simulink model "DFIGPI_by_indraneel_saki"  (Simulink 10.0)
settings: Solver=ode23t  StartTime=0.0  StopTime=1.5  RelTol=1e-3  EnableMultiTasking=on
libraries: simulink x3, powerlib_extras x1, DRlib x1, powerlib x1
settings Model: Creator=SRIDHAR  LastModifiedBy=bhisma
settings SolverCC: ZeroCrossControl=DisableAll
settings DataIOCC: LimitDataPoints=on  SignalLoggingSaveFormat=ModelDataLogs
settings OptimizationCC: ExpressionDepthLimit=2147483647  InitFltsAndDblsToZero=on
settings DebuggingCC: SaveWithParameterizedLinksMsg=none  SignalResolutionControl=TryResolveAllWithWarning  SolverPrmCheckMsg=warning  FcnCallInpInsideContextMsg=warning  StateNameClashWarn=warning
settings GRTTargetCC: TargetFcnLib=ansi_tfl_tmw.mat  GeneratePreprocessorConditionals=Disable all
settings ConfigComp: CovExternalEMLEnable=off
settings SimscapeCC: SimscapeNormalizeSystem=off

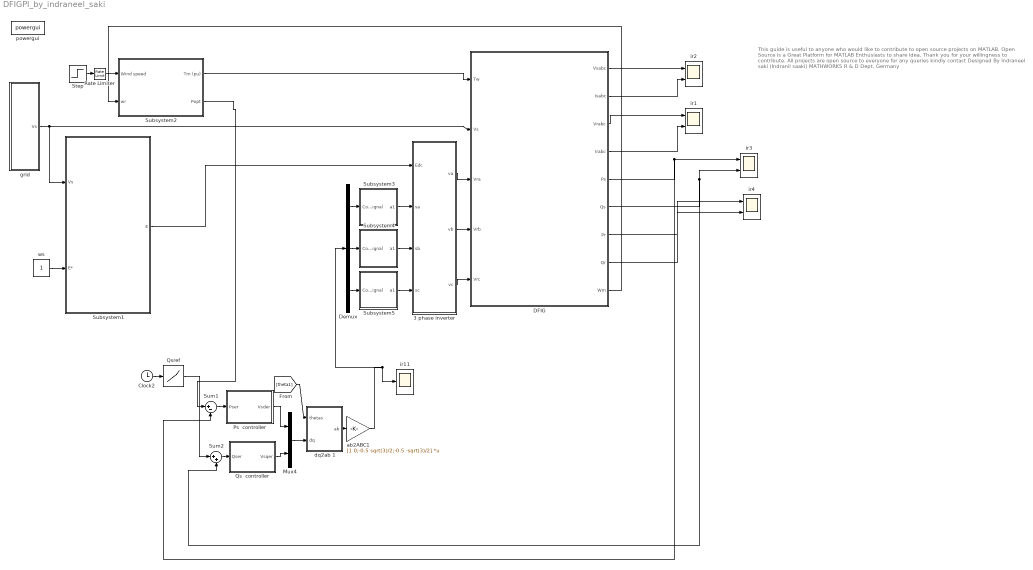
== system DFIGPI_by_indraneel_saki ==
  note: This guide is useful to anyone who would like to contribute to open source projects on MATLAB.
      | Open Source is a Great Platform for MATLAB Enthusiasts to share idea. Thank you for your willingness to contribute.
      | All projects are open source to everyone for any queries kindly contact
      | Designed By Indraneel saki (Indranil saaki)
      | MATHWORKS R & D Dept.
      | Germany
  3 phase inverter : Subsystem
  Clock2 : Clock
  DFIG : Subsystem
      mask Display: disp('DOUBLY FED\nINDUCTION\nGENERTATOR')
  Demux : Demux  Outputs=3
  Mux4 : Mux  Inputs=2
  Ps  controller : Subsystem  mask{Kp=0.07, Ki=10, sat=10}
      mask prompts: Kp "Proportional gain (Kp)"; Ki "Integral gain (Ki)"; sat "Saturation limit [pu]"
      mask help: Proportional-Integral Speed Controller
  Qs  controller : Subsystem  mask{Kp=0.07, Ki=10, sat=1000}
      mask prompts: Kp "Proportional gain (Kp)"; Ki "Integral gain (Ki)"; sat "Saturation limit [pu]"
      mask help: Proportional-Integral Speed Controller
  Qsref : Lookup  InputValues=[0 4 4 5]  Table=[1 1 4 1]  SaturateOnIntegerOverflow=on
  Rate Limiter : RateLimiter
  Step : Step  Time=5  Before=8  After=14  SampleTime=0
  Subsystem1 : Subsystem
      mask Display: disp('front end \n converter ')
  Subsystem2 : Subsystem  mask{speed_power=[0 0; 0.24 0.007; 0.36 0.024; 0.6 0.112; 0.96 0.46; 1.2 0.898; 1.5 0.898], speed_ABCD=[0.7 0.71 1.2 1.21], power_slew_rate=1, pitch_rate=2, pitch_max=45, pitch_gain=500}
      mask prompts: speed_power "Electric power-speed characteristic: [wr1(pu) p1(pu); wr2(pu) p2(pu); ... ]"; speed_ABCD "Tracking characteristic speeds: [speed_A(pu) ... speed_D(pu)]"; power_slew_rate "Maximum rate of change of reference power (p.u./s):"; pitch_rate "Maximum rate of change of pitch angle (deg/s):"; pitch_max "Maximum pitch angle (deg):"; pitch_gain "Pitch angle controller gain [Kp]:"
      mask Display: disp('Wind\nTurbine')
  Subsystem3 : Subsystem  mask{fs=2000}
      mask prompts: fs "Switching Frequency"
  Subsystem4 : Subsystem  mask{fs=2000}
      mask prompts: fs "Switching Frequency"
  Subsystem5 : Subsystem  mask{fs=2000}
      mask prompts: fs "Switching Frequency"
  Sum1 : Sum  Inputs=|+-  SaturateOnIntegerOverflow=on
  Sum2 : Sum  Inputs=|++  SaturateOnIntegerOverflow=on
  ab2ABC1 : Gain  Gain=[1 0;-0.5 sqrt(3)/2;-0.5 -sqrt(3)/2]  Multiplication=Matrix(K*u)  SaturateOnIntegerOverflow=on  OutDataTypeStr=Inherit: Same as input  ParamDataTypeStr=Inherit: Same as input
  dq2ab 1 : Subsystem
  grid : Subsystem
      mask Display: disp('GRID')
  ir{1..4} (4 alike) : Scope  NumInputPorts=2
  ir11 : Scope
  powergui : powerlib/powergui  SystemSampleTime=-1  SimulationMode=Continuous  SampleTime=50e-6  frequency=60  SPID=off  DisableSnubberDevices=off  DisableRonSwitches=off  DisableVfSwitches=off  SwTol=0  Interpol=off  frequencyindice=0  echomessages=off  HookPort=off  DisplayEquations=off  FunctionMessages=off  EnableUseOfTLC=off  x0status=blocks  RestoreLinks=warning  Frange=[0:2:500]  Ylog=off  Xlog=on  ShowGrid=off  save=off  variable=ZData  ZoomFFT=on  StartTime=0.0  cycles=1  DisplayStyle=1  fundamental=60  FreqAxis=off  MaxFrequency=1000  frequencyindicesteady=1  RmsSteady=1  display=off  Ts=0  methode=off
      settings: SourceProductName=Simscape Electrical
  ws : Constant
  wires:
  grid/1(Vs) -> Subsystem1/1(Vs), DFIG/2(Vs)
  3 phase inverter/1(va) -> DFIG/3(Vra)
  3 phase inverter/2(vb) -> DFIG/4(Vrb)
  3 phase inverter/3(vc) -> DFIG/5(Vrc)
  DFIG/1(Vsabc) -> ir2/1
  DFIG/2(Isabc) -> ir2/2
  DFIG/3(Vrabc) -> ir1/1
  DFIG/4(Irabc) -> ir1/2
  Demux/3 -> Subsystem5/1(Control signal)
  Demux/1 -> Subsystem3/1(Control signal)
  Demux/2 -> Subsystem4/1(Control signal)
  Subsystem1/1(E) -> 3 phase inverter/1(Edc)
  ws/1 -> Subsystem1/2("E* ")
  DFIG/7(Pr) -> ir4/1
  DFIG/8(Qr) -> ir4/2
  DFIG/5(Ps) -> Sum1/2, ir3/1
  DFIG/6(Qs) -> Sum2/2, ir3/2
  Qsref/1 -> Sum2/1
  Subsystem2/1(Tm (pu)) -> DFIG/1(Tw)
  Subsystem2/2(Popt) -> Sum1/1
  DFIG/9(Wm) -> Subsystem2/2(wr)
  Step/1 -> Rate Limiter/1
  Sum1/1 -> Ps  controller/1(Pser)
  Sum2/1 -> Qs  controller/1(Qser)
  Ps  controller/1(Vsder) -> Mux4/1
  Qs  controller/1(Vsqer) -> Mux4/2
  Mux4/1 -> dq2ab 1/2(dq)
  dq2ab 1/1(ab) -> ab2ABC1/1
  ab2ABC1/1 -> Demux/1, ir11/1
  [theta1] -> dq2ab 1/1(thetas)
  Clock2/1 -> Qsref/1
  Subsystem3/1(a1) -> 3 phase inverter/2(sa)
  Subsystem4/1(a1) -> 3 phase inverter/3(sb)
  Subsystem5/1(a1) -> 3 phase inverter/4(sc)
  Rate Limiter/1 -> Subsystem2/1("Wind speed ")

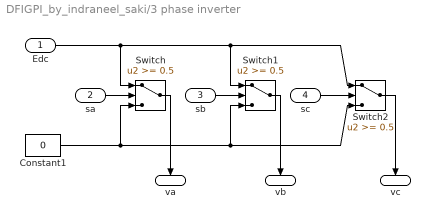
== system DFIGPI_by_indraneel_saki/3 phase inverter ==
  Edc : Inport
  sa : Inport  Port=2
  sb : Inport  Port=3
  sc : Inport  Port=4
  Constant1 : Constant  Value=0
  Switch : Switch  Threshold=0.5  SaturateOnIntegerOverflow=on  InputSameDT=on
  Switch1 : Switch  Threshold=0.5  SaturateOnIntegerOverflow=on  InputSameDT=on
  Switch2 : Switch  Threshold=0.5  SaturateOnIntegerOverflow=on  InputSameDT=on
  va : Outport  InitialOutput=0
  vb : Outport  Port=2  InitialOutput=0
  vc : Outport  Port=3  InitialOutput=0
  wires:
  Switch1/1 -> vb/1
  Switch2/1 -> vc/1
  sc/1 -> Switch2/2
  sb/1 -> Switch1/2
  Switch/1 -> va/1
  sa/1 -> Switch/2
  Constant1/1 -> Switch2/3, Switch1/3, Switch/3
  Edc/1 -> Switch2/1, Switch1/1, Switch/1

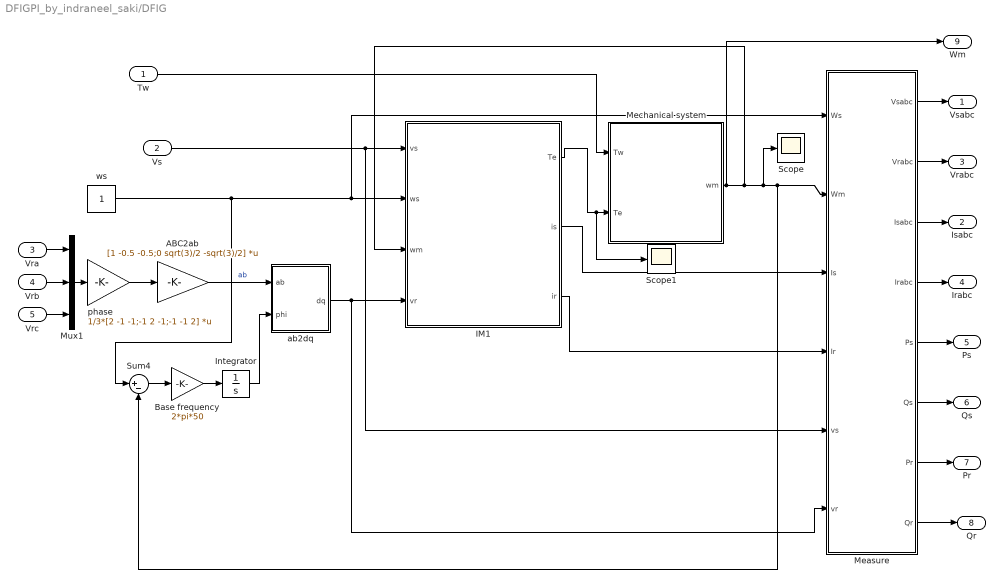
== system DFIGPI_by_indraneel_saki/DFIG ==
  Tw : Inport
  Vs : Inport  Port=2
  Vra : Inport  Port=3
  Vrb : Inport  Port=4
  Vrc : Inport  Port=5
  ABC2ab : Gain  Gain=[1 -0.5 -0.5;0 sqrt(3)/2 -sqrt(3)/2]  Multiplication=Matrix(K*u)  SaturateOnIntegerOverflow=on  OutDataTypeStr=Inherit: Same as input  ParamDataTypeStr=Inherit: Same as input
  Base frequency : Gain  Gain=2*pi*50  SaturateOnIntegerOverflow=on  OutDataTypeStr=Inherit: Same as input  ParamDataTypeStr=Inherit: Same as input
  IM1 : Subsystem  mask{Rs=0.05, Lsl=0.5, Rr=0.02, Lm=5, Lrl=0.1, wo=100*pi}
      mask prompts: Rs "Stator resistance [pu]"; Lsl "Stator leakage inductance [pu]"; Rr "Rotor resistance [pu]"; Lm "Magnetizing inductance [pu]"; Lrl "Rotor leakage inductance [pu]"; wo "base frequency [rad/s]"
      mask Display: disp('DOUBLY FED\nINDUCTION GENERTATOR')
  Integrator : Integrator
  Measure : Subsystem
  Mechanical system : Subsystem  mask{Hw=2.5, Hg=0.5, Km=.4}
      mask prompts: Hw "Turbine inertia constant [s]"; Hg "Generator inertia constant [s]"; Km "Shaft compliance constant [pu/rad]"
      mask Display: disp('Mechanical\nSystem')
  Mux1 : Mux  Inputs=3
  Scope : Scope
  Scope1 : Scope
  Sum4 : Sum  Inputs=|+-  SaturateOnIntegerOverflow=on  InputSameDT=on  OutDataTypeStr=Inherit: Same as first input
  ab2dq : Subsystem
  phase : Gain  Gain=1/3*[2 -1 -1;-1 2 -1;-1 -1 2]  Multiplication=Matrix(K*u)  SaturateOnIntegerOverflow=on  OutDataTypeStr=Inherit: Same as input  ParamDataTypeStr=Inherit: Same as input
  ws : Constant
  Vsabc : Outport
  Isabc : Outport  Port=2
  Vrabc : Outport  Port=3
  Irabc : Outport  Port=4
  Ps : Outport  Port=5
  Qs : Outport  Port=6
  Pr : Outport  Port=7
  Qr : Outport  Port=8
  Wm : Outport  Port=9
  wires:
  Vra/1 -> Mux1/1
  Vrb/1 -> Mux1/2
  Vrc/1 -> Mux1/3
  Mux1/1 -> phase/1
  Measure/1(Vsabc) -> Vsabc/1
  Measure/2(Vrabc) -> Vrabc/1
  Measure/3(Isabc) -> Isabc/1
  Measure/4(Irabc) -> Irabc/1
  Measure/5(Ps) -> Ps/1
  Measure/6(Qs) -> Qs/1
  phase/1 -> ABC2ab/1
  Mechanical system/1(wm) -> Wm/1, IM1/3(wm), Measure/2(Wm), Sum4/2, Scope/1
  IM1/1(Te) -> Mechanical system/2(Te), Scope1/1
  Tw/1 -> Mechanical system/1(Tw)
  ws/1 -> Measure/1(Ws), IM1/2(ws), Sum4/1
  Vs/1 -> IM1/1(vs), Measure/5(vs)
  IM1/2(is) -> Measure/3(Is)
  IM1/3(ir) -> Measure/4(Ir)
  Measure/7(Pr) -> Pr/1
  Measure/8(Qr) -> Qr/1
  ABC2ab/1 -> ab2dq/1(ab)  "ab"
  Base frequency/1 -> Integrator/1
  Integrator/1 -> ab2dq/2(phi)
  Sum4/1 -> Base frequency/1
  ab2dq/1(dq) -> IM1/4(vr), Measure/6(vr)

== system DFIGPI_by_indraneel_saki/Ps  controller ==
  Pser : Inport
  Gain : Gain  Gain=Ki  SaturateOnIntegerOverflow=on  OutDataTypeStr=Inherit: Same as input  ParamDataTypeStr=Inherit: Same as input
  Gain1 : Gain  Gain=Kp  SaturateOnIntegerOverflow=on  OutDataTypeStr=Inherit: Same as input  ParamDataTypeStr=Inherit: Same as input
  Integrator : Integrator  LimitOutput=on  UpperSaturationLimit=sat  LowerSaturationLimit=-sat
  Saturation : Saturate  UpperLimit=sat  LowerLimit=-sat
  Sum : Sum  SaturateOnIntegerOverflow=on  InputSameDT=on  OutDataTypeStr=Inherit: Same as first input
  Vsder : Outport  InitialOutput=0
  wires:
  Integrator/1 -> Sum/2
  Gain1/1 -> Sum/1
  Gain/1 -> Integrator/1
  Pser/1 -> Gain/1, Gain1/1
  Sum/1 -> Saturation/1
  Saturation/1 -> Vsder/1

== system DFIGPI_by_indraneel_saki/Qs  controller ==
  Qser : Inport
  Gain : Gain  Gain=Ki  SaturateOnIntegerOverflow=on  OutDataTypeStr=Inherit: Same as input  ParamDataTypeStr=Inherit: Same as input
  Gain1 : Gain  Gain=Kp  SaturateOnIntegerOverflow=on  OutDataTypeStr=Inherit: Same as input  ParamDataTypeStr=Inherit: Same as input
  Integrator : Integrator  LimitOutput=on  UpperSaturationLimit=sat  LowerSaturationLimit=-sat
  Saturation : Saturate  UpperLimit=sat  LowerLimit=-sat
  Sum : Sum  SaturateOnIntegerOverflow=on  InputSameDT=on  OutDataTypeStr=Inherit: Same as first input
  Vsqer : Outport  InitialOutput=0
  wires:
  Saturation/1 -> Vsqer/1
  Sum/1 -> Saturation/1
  Qser/1 -> Gain1/1, Gain/1
  Gain/1 -> Integrator/1
  Gain1/1 -> Sum/1
  Integrator/1 -> Sum/2

== system DFIGPI_by_indraneel_saki/Subsystem1 ==
  Vs : Inport
  "E* " : Inport  Port=2
  Ps  controller : Subsystem  mask{Kp=0.07, Ki=10, sat=1000}
      mask prompts: Kp "Proportional gain (Kp)"; Ki "Integral gain (Ki)"; sat "Saturation limit [pu]"
      mask help: Proportional-Integral Speed Controller
  Subsystem : Subsystem
      mask Display: disp('INVERTER')
  Sum : Sum  Inputs=|+-
  Transfer Fcn : TransferFcn  Denominator=[2.4e-6 0]
  E : Outport
  wires:
  Transfer Fcn/1 -> Sum/2, E/1
  "E* "/1 -> Sum/1, Subsystem/2("E* ")
  Sum/1 -> Ps  controller/1(Pser)
  Subsystem/1(Ios) -> Transfer Fcn/1
  Vs/1 -> Subsystem/1(Vs)
  Ps  controller/1(Vsder) -> Subsystem/3(Id)

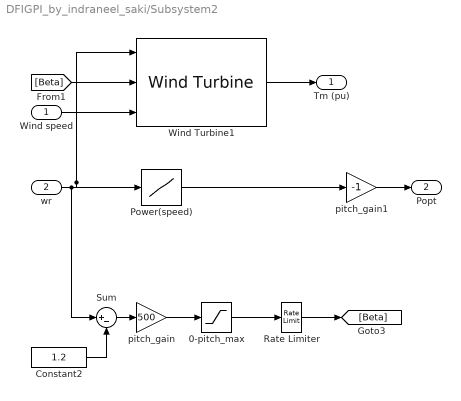
== system DFIGPI_by_indraneel_saki/Subsystem2 ==
  "Wind speed " : Inport
  wr : Inport  Port=2
  0-pitch_max : Saturate  UpperLimit=pitch_max  LowerLimit=0
  Constant2 : Constant  Value=1.2
  Power(speed) : Lookup  InputValues=speed_power(:,1)  Table=speed_power(:,2)  SaturateOnIntegerOverflow=on
  "Rate Limiter   " : RateLimiter  RisingSlewLimit=pitch_rate  FallingSlewLimit=-pitch_rate
  Sum : Sum  Inputs=|+-  SaturateOnIntegerOverflow=on
  Wind Turbine1 : DRlib/Wind Generation/Wind Turbine  SystemSampleTime=-1  Pnom=1.5e6  Pelec_base=1.5e6/0.9  wind_base=12  P_wind_base=0.73  speed_nom=1.2  pitch_angle=0  DisplayTurbChar=off  c1_c6="[0.51763          116          0.4            5           21     0.006795]"  cp_nom=0.48  lambda_nom=8.1
      settings: SourceProductName=Simscape Electrical  SourceProductBaseCode=PS
  pitch_gain : Gain  Gain=500  SaturateOnIntegerOverflow=on  OutDataTypeStr=Inherit: Same as input  ParamDataTypeStr=Inherit: Same as input
  pitch_gain1 : Gain  Gain=-1  SaturateOnIntegerOverflow=on  OutDataTypeStr=Inherit: Same as input  ParamDataTypeStr=Inherit: Same as input
  Tm (pu) : Outport
  Popt : Outport  Port=2
  wires:
  wr/1 -> Sum/1, Wind Turbine1/1, Power(speed)/1
  pitch_gain/1 -> 0-pitch_max/1
  Sum/1 -> pitch_gain/1
  Constant2/1 -> Sum/2
  [Beta] -> Wind Turbine1/2
  Wind Turbine1/1 -> Tm (pu)/1
  "Wind speed "/1 -> Wind Turbine1/3
  Power(speed)/1 -> pitch_gain1/1
  pitch_gain1/1 -> Popt/1
  "Rate Limiter   "/1 -> [Beta]
  0-pitch_max/1 -> "Rate Limiter   "/1

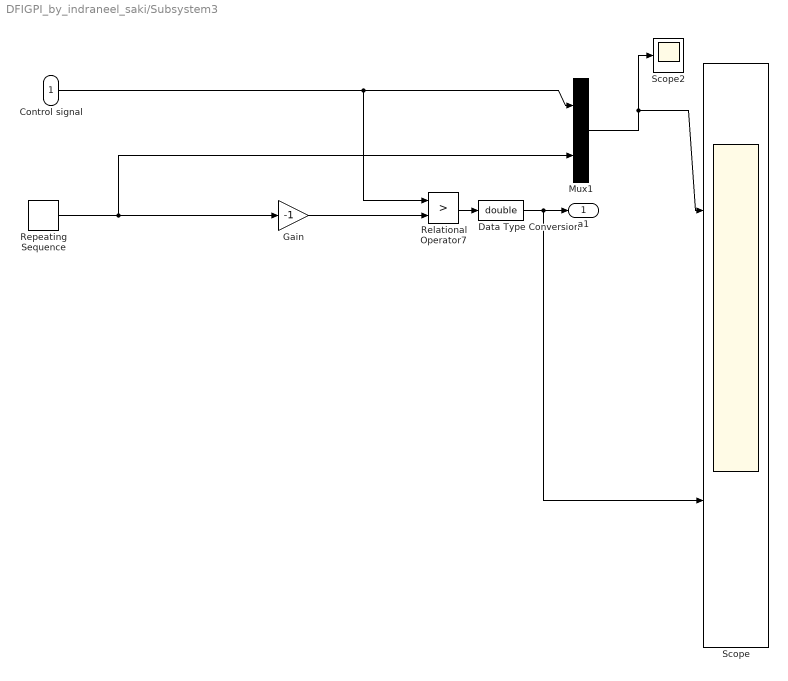
== system DFIGPI_by_indraneel_saki/Subsystem3 ==
  Control signal : Inport
  Data Type Conversion : DataTypeConversion  OutDataTypeStr=double
  Gain : Gain  Gain=-1
  Mux1 : Mux  Inputs=2
  Relational Operator7 : RelationalOperator  Operator=>  OutDataTypeStr=uint(8)  RndMeth=Nearest
  Repeating Sequence : simulink/Sources/Repeating Sequence  SystemSampleTime=-1  rep_seq_t=[0 (1/fs)/2 1/fs]  rep_seq_y=[1 -1 1 ]
  Scope : Scope  NumInputPorts=2
  Scope2 : Scope
  a1 : Outport
  wires:
  Repeating Sequence/1 -> Mux1/2, Gain/1
  Relational Operator7/1 -> Data Type Conversion/1
  Control signal/1 -> Mux1/1, Relational Operator7/1
  Data Type Conversion/1 -> a1/1, Scope/2
  Gain/1 -> Relational Operator7/2
  Mux1/1 -> Scope/1, Scope2/1

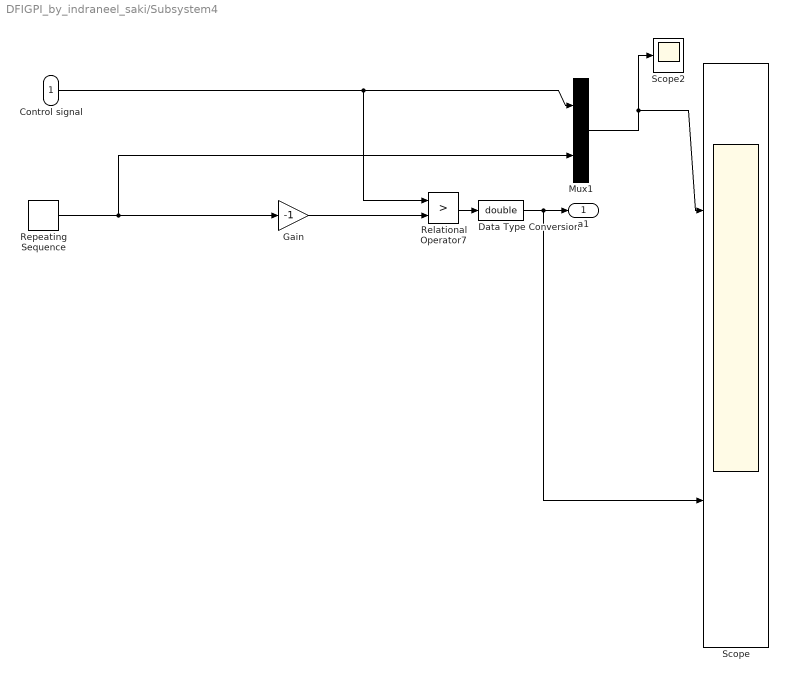
== system DFIGPI_by_indraneel_saki/Subsystem4 ==
  Control signal : Inport
  Data Type Conversion : DataTypeConversion  OutDataTypeStr=double
  Gain : Gain  Gain=-1
  Mux1 : Mux  Inputs=2
  Relational Operator7 : RelationalOperator  Operator=>  OutDataTypeStr=uint(8)  RndMeth=Nearest
  Repeating Sequence : simulink/Sources/Repeating Sequence  SystemSampleTime=-1  rep_seq_t=[0 (1/fs)/2 1/fs]  rep_seq_y=[1 -1 1 ]
  Scope : Scope  NumInputPorts=2
  Scope2 : Scope
  a1 : Outport
  wires:
  Mux1/1 -> Scope2/1, Scope/1
  Gain/1 -> Relational Operator7/2
  Data Type Conversion/1 -> Scope/2, a1/1
  Control signal/1 -> Relational Operator7/1, Mux1/1
  Relational Operator7/1 -> Data Type Conversion/1
  Repeating Sequence/1 -> Gain/1, Mux1/2

== system DFIGPI_by_indraneel_saki/Subsystem5 ==
  Control signal : Inport
  Data Type Conversion : DataTypeConversion  OutDataTypeStr=double
  Gain : Gain  Gain=-1
  Mux1 : Mux  Inputs=2
  Relational Operator7 : RelationalOperator  Operator=>  OutDataTypeStr=uint(8)  RndMeth=Nearest
  Repeating Sequence : simulink/Sources/Repeating Sequence  SystemSampleTime=-1  rep_seq_t=[0 (1/fs)/2 1/fs]  rep_seq_y=[1 -1 1 ]
  Scope : Scope  NumInputPorts=2
  Scope2 : Scope
  a1 : Outport
  wires:
  Repeating Sequence/1 -> Mux1/2, Gain/1
  Relational Operator7/1 -> Data Type Conversion/1
  Control signal/1 -> Mux1/1, Relational Operator7/1
  Data Type Conversion/1 -> a1/1, Scope/2
  Gain/1 -> Relational Operator7/2
  Mux1/1 -> Scope/1, Scope2/1

== system DFIGPI_by_indraneel_saki/dq2ab 1 ==
  thetas : Inport
  dq : Inport  Port=2
  Fcn : Fcn  Expr=u(1)*cos(u(3))-u(2)*sin(u(3))
  Fcn1 : Fcn  Expr=u(1)*sin(u(3))+u(2)*cos(u(3))
  Mux3 : Mux  Inputs=2
  Mux4 : Mux  Inputs=2
  Mux5 : Mux  Inputs=2
  ab : Outport
  wires:
  Mux5/1 -> ab/1
  Fcn/1 -> Mux5/1
  Fcn1/1 -> Mux5/2
  thetas/1 -> Mux4/2, Mux3/2
  dq/1 -> Mux4/1, Mux3/1
  Mux4/1 -> Fcn1/1
  Mux3/1 -> Fcn/1

== system DFIGPI_by_indraneel_saki/grid ==
  note: Vds
  note: Vqs
  Mux3 : Mux  Inputs=2
  Vds : Constant
  vqs : Constant  Value=0
  Vs : Outport
  wires:
  Mux3/1 -> Vs/1
  Vds/1 -> Mux3/1
  vqs/1 -> Mux3/2

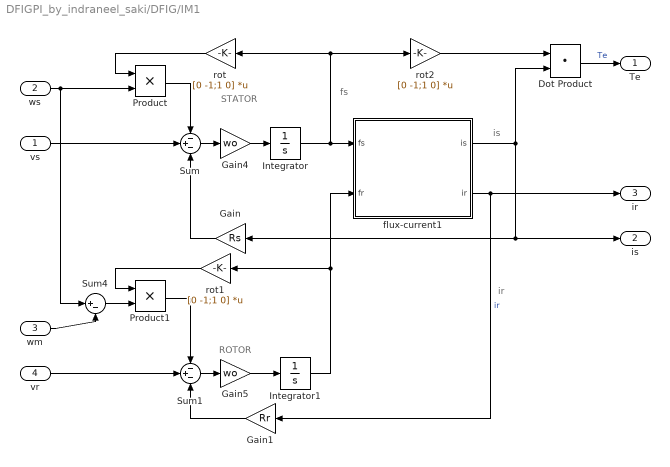
== system DFIGPI_by_indraneel_saki/DFIG/IM1 ==
  note: fs
  note: is
  note: ir
  note: ROTOR
  note: STATOR
  vs : Inport
  ws : Inport  Port=2
  wm : Inport  Port=3
  vr : Inport  Port=4
  Dot Product : DotProduct  InputSameDT=on  OutDataTypeStr=Inherit: Inherit via internal rule
  Gain : Gain  Gain=Rs  SaturateOnIntegerOverflow=on  OutDataTypeStr=Inherit: Same as input  ParamDataTypeStr=Inherit: Same as input
  Gain1 : Gain  Gain=Rr  SaturateOnIntegerOverflow=on  OutDataTypeStr=Inherit: Same as input  ParamDataTypeStr=Inherit: Same as input
  Gain4 : Gain  Gain=wo  SaturateOnIntegerOverflow=on  OutDataTypeStr=Inherit: Same as input  ParamDataTypeStr=Inherit: Same as input
  Gain5 : Gain  Gain=wo  SaturateOnIntegerOverflow=on  OutDataTypeStr=Inherit: Same as input  ParamDataTypeStr=Inherit: Same as input
  Integrator : Integrator
  Integrator1 : Integrator
  Product : Product  SaturateOnIntegerOverflow=on  InputSameDT=on  OutDataTypeStr=Inherit: Same as first input
  Product1 : Product  SaturateOnIntegerOverflow=on  InputSameDT=on  OutDataTypeStr=Inherit: Same as first input
  Sum : Sum  Inputs=-+-  SaturateOnIntegerOverflow=on  InputSameDT=on  OutDataTypeStr=Inherit: Same as first input
  Sum1 : Sum  Inputs=-+-  SaturateOnIntegerOverflow=on  InputSameDT=on  OutDataTypeStr=Inherit: Same as first input
  Sum4 : Sum  Inputs=|+-  SaturateOnIntegerOverflow=on  InputSameDT=on  OutDataTypeStr=Inherit: Same as first input
  flux-current1 : Subsystem
  rot : Gain  Gain=[0 -1;1 0]  Multiplication=Matrix(K*u)  SaturateOnIntegerOverflow=on  OutDataTypeStr=Inherit: Same as input  ParamDataTypeStr=Inherit: Same as input
  rot1 : Gain  Gain=[0 -1;1 0]  Multiplication=Matrix(K*u)  SaturateOnIntegerOverflow=on  OutDataTypeStr=Inherit: Same as input  ParamDataTypeStr=Inherit: Same as input
  rot2 : Gain  Gain=[0 -1;1 0]  Multiplication=Matrix(K*u)  SaturateOnIntegerOverflow=on  OutDataTypeStr=Inherit: Same as input  ParamDataTypeStr=Inherit: Same as input
  Te : Outport
  is : Outport  Port=2
  ir : Outport  Port=3
  wires:
  Gain/1 -> Sum/3
  Gain1/1 -> Sum1/3
  flux-current1/2(ir) -> Gain1/1, ir/1  "ir"
  Integrator/1 -> flux-current1/1(fs), rot/1, rot2/1
  Integrator1/1 -> flux-current1/2(fr), rot1/1
  Product1/1 -> Sum1/1
  rot1/1 -> Product1/1
  Product/1 -> Sum/1
  rot/1 -> Product/1
  rot2/1 -> Dot Product/1
  Sum4/1 -> Product1/2
  Sum/1 -> Gain4/1
  Gain4/1 -> Integrator/1
  Sum1/1 -> Gain5/1
  Gain5/1 -> Integrator1/1
  flux-current1/1(is) -> Gain/1, is/1, Dot Product/2
  Dot Product/1 -> Te/1  "Te"
  vs/1 -> Sum/2
  ws/1 -> Product/2, Sum4/1
  wm/1 -> Sum4/2
  vr/1 -> Sum1/2

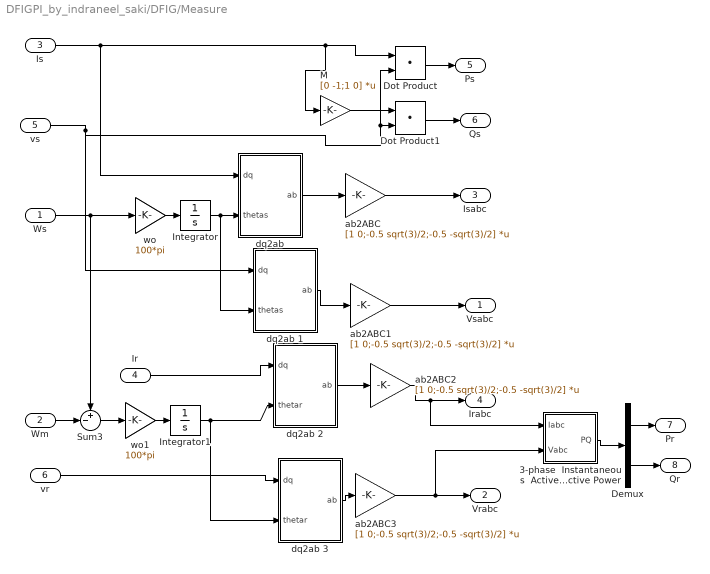
== system DFIGPI_by_indraneel_saki/DFIG/Measure ==
  Ws : Inport
  Wm : Inport  Port=2
  Is : Inport  Port=3
  Ir : Inport  Port=4
  vs : Inport  Port=5
  vr : Inport  Port=6
  3-phase  Instantaneous  Active & Reactive Power : Subsystem  AncestorBlock=|  DialogController=PMDialogs.PMDefaultMaskDlg  mask(3-phase instantaneous active and reactive power){}
      | powerlib_extras/Measurements/3-phase 
      | Instantaneous 
      | Active & Reactive Power
      mask help:
      | This block computes the 3-phase instantaneous active (P) and reactive (Q) power associated with a periodic set of 3-phase voltages and currents.
      | Note: Result for the instantaneous reactive power (Q) is accurate only for balanced and harmonic-free 3-phase quantities (voltages and currents).
      |
      | Input 1: Vectorized 3-phase  instantaneous voltage (Vabc)
      | Input 2: Vectorized 3-phase instantaneous current (Iabc)
      | Output : Computed PQ vector [P(W) Q(var)]. Current flowing into an RL circuit will produce  positive active and reactive power.
      mask init:
      | power_initmask();
      mask Help: This block is part of a subset of blocks in the Extras library that does not have documentation associated with it, other than the block mask description.
  Demux : Demux  Outputs=2
  Dot Product : DotProduct  InputSameDT=on  OutDataTypeStr=Inherit: Inherit via internal rule
  Dot Product1 : DotProduct  InputSameDT=on  OutDataTypeStr=Inherit: Inherit via internal rule
  Integrator : Integrator
  Integrator1 : Integrator
  M : Gain  Gain=[0 -1;1 0]  Multiplication=Matrix(K*u)  SaturateOnIntegerOverflow=on  OutDataTypeStr=Inherit: Same as input  ParamDataTypeStr=Inherit: Same as input
  Sum3 : Sum  Inputs=+-|  SaturateOnIntegerOverflow=on
  ab2ABC{,1..3} (4 alike) : Gain  Gain=[1 0;-0.5 sqrt(3)/2;-0.5 -sqrt(3)/2]  Multiplication=Matrix(K*u)  SaturateOnIntegerOverflow=on  OutDataTypeStr=Inherit: Same as input  ParamDataTypeStr=Inherit: Same as input
  "dq2ab " : Subsystem
  dq2ab 1 : Subsystem
  dq2ab 2 : Subsystem
  dq2ab 3 : Subsystem
  wo : Gain  Gain=100*pi  SaturateOnIntegerOverflow=on  OutDataTypeStr=Inherit: Same as input  ParamDataTypeStr=Inherit: Same as input
  wo1 : Gain  Gain=100*pi  SaturateOnIntegerOverflow=on  OutDataTypeStr=Inherit: Same as input  ParamDataTypeStr=Inherit: Same as input
  Vsabc : Outport
  Vrabc : Outport  Port=2
  Isabc : Outport  Port=3
  Irabc : Outport  Port=4
  Ps : Outport  Port=5
  Qs : Outport  Port=6
  Pr : Outport  Port=7
  Qr : Outport  Port=8
  wires:
  Is/1 -> "dq2ab "/1(dq), M/1, Dot Product/1
  vs/1 -> dq2ab 1/1(dq), Dot Product/2, Dot Product1/2
  Ir/1 -> dq2ab 2/1(dq)
  vr/1 -> dq2ab 3/1(dq)
  "dq2ab "/1(ab) -> ab2ABC/1
  ab2ABC/1 -> Isabc/1
  wo/1 -> Integrator/1
  Integrator/1 -> "dq2ab "/2(thetas), dq2ab 1/2(thetas)
  Ws/1 -> Sum3/1, wo/1
  dq2ab 1/1(ab) -> ab2ABC1/1
  ab2ABC1/1 -> Vsabc/1
  Wm/1 -> Sum3/2
  Sum3/1 -> wo1/1
  wo1/1 -> Integrator1/1
  dq2ab 2/1(ab) -> ab2ABC2/1
  ab2ABC2/1 -> Irabc/1, 3-phase  Instantaneous  Active & Reactive Power/1(Iabc)
  Integrator1/1 -> dq2ab 2/2(thetar), dq2ab 3/2(thetar)
  dq2ab 3/1(ab) -> ab2ABC3/1
  ab2ABC3/1 -> Vrabc/1, 3-phase  Instantaneous  Active & Reactive Power/2(Vabc)
  Dot Product/1 -> Ps/1
  Dot Product1/1 -> Qs/1
  M/1 -> Dot Product1/1
  3-phase  Instantaneous  Active & Reactive Power/1(PQ) -> Demux/1
  Demux/1 -> Pr/1
  Demux/2 -> Qr/1

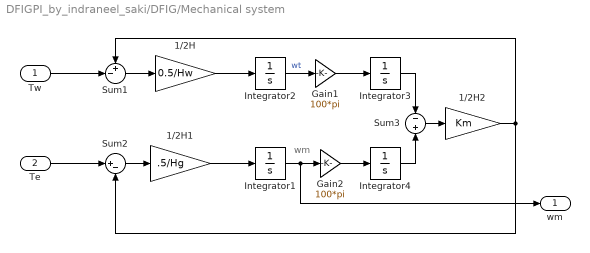
== system DFIGPI_by_indraneel_saki/DFIG/Mechanical system ==
  note: wm
  Tw : Inport
  Te : Inport  Port=2
  1/2H : Gain  Gain=0.5/Hw  SaturateOnIntegerOverflow=on  OutDataTypeStr=Inherit: Same as input  ParamDataTypeStr=Inherit: Same as input
  1/2H1 : Gain  Gain=.5/Hg  SaturateOnIntegerOverflow=on  OutDataTypeStr=Inherit: Same as input  ParamDataTypeStr=Inherit: Same as input
  1/2H2 : Gain  Gain=Km  SaturateOnIntegerOverflow=on  OutDataTypeStr=Inherit: Same as input  ParamDataTypeStr=Inherit: Same as input
  Gain1 : Gain  Gain=100*pi  SaturateOnIntegerOverflow=on  OutDataTypeStr=Inherit: Same as input  ParamDataTypeStr=Inherit: Same as input
  Gain2 : Gain  Gain=100*pi  SaturateOnIntegerOverflow=on  OutDataTypeStr=Inherit: Same as input  ParamDataTypeStr=Inherit: Same as input
  Integrator{1..4} (4 alike) : Integrator
  Sum1 : Sum  Inputs=+-|  SaturateOnIntegerOverflow=on
  Sum2 : Sum  Inputs=|+-  SaturateOnIntegerOverflow=on
  Sum3 : Sum  Inputs=-+  SaturateOnIntegerOverflow=on
  wm : Outport
  wires:
  Tw/1 -> Sum1/2
  Sum1/1 -> 1/2H/1
  Te/1 -> Sum2/1
  1/2H/1 -> Integrator2/1
  Sum2/1 -> 1/2H1/1
  1/2H1/1 -> Integrator1/1
  Integrator3/1 -> Sum3/1
  Sum3/1 -> 1/2H2/1
  1/2H2/1 -> Sum1/1, Sum2/2
  Gain1/1 -> Integrator3/1
  Integrator2/1 -> Gain1/1  "wt"
  Gain2/1 -> Integrator4/1
  Integrator4/1 -> Sum3/2
  Integrator1/1 -> Gain2/1, wm/1

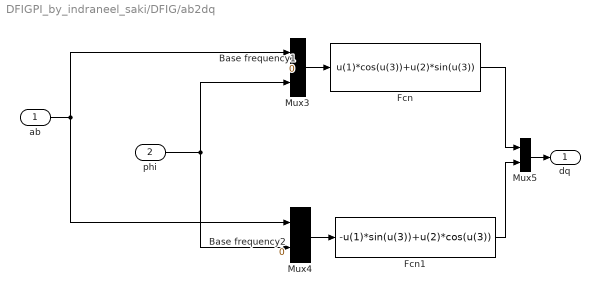
== system DFIGPI_by_indraneel_saki/DFIG/ab2dq ==
  ab : Inport
  phi : Inport  Port=2
  Base frequency1 : Gain  Gain=0  SaturateOnIntegerOverflow=on  OutDataTypeStr=Inherit: Same as input  ParamDataTypeStr=Inherit: Same as input
  Base frequency2 : Gain  Gain=0  SaturateOnIntegerOverflow=on  OutDataTypeStr=Inherit: Same as input  ParamDataTypeStr=Inherit: Same as input
  Fcn : Fcn  Expr=u(1)*cos(u(3))+u(2)*sin(u(3))
  Fcn1 : Fcn  Expr=-u(1)*sin(u(3))+u(2)*cos(u(3))
  Mux3 : Mux  Inputs=2
  Mux4 : Mux  Inputs=2
  Mux5 : Mux  Inputs=2
  dq : Outport
  wires:
  Mux3/1 -> Fcn/1
  Mux4/1 -> Fcn1/1
  ab/1 -> Mux3/1, Mux4/1
  Fcn1/1 -> Mux5/2
  Fcn/1 -> Mux5/1
  Mux5/1 -> dq/1
  phi/1 -> Base frequency1/1, Base frequency2/1
  Base frequency1/1 -> Mux3/2
  Base frequency2/1 -> Mux4/2

== system DFIGPI_by_indraneel_saki/Subsystem1/Ps  controller ==
  Pser : Inport
  Gain : Gain  Gain=Ki  SaturateOnIntegerOverflow=on  OutDataTypeStr=Inherit: Same as input  ParamDataTypeStr=Inherit: Same as input
  Gain1 : Gain  Gain=Kp  SaturateOnIntegerOverflow=on  OutDataTypeStr=Inherit: Same as input  ParamDataTypeStr=Inherit: Same as input
  Integrator : Integrator  LimitOutput=on  UpperSaturationLimit=sat  LowerSaturationLimit=-sat
  Saturation : Saturate  UpperLimit=sat  LowerLimit=-sat
  Sum : Sum  SaturateOnIntegerOverflow=on  InputSameDT=on  OutDataTypeStr=Inherit: Same as first input
  Vsder : Outport  InitialOutput=0
  wires:
  Integrator/1 -> Sum/2
  Gain1/1 -> Sum/1
  Pser/1 -> Gain/1, Gain1/1
  Sum/1 -> Saturation/1
  Saturation/1 -> Vsder/1
  Gain/1 -> Integrator/1

== system DFIGPI_by_indraneel_saki/Subsystem1/Subsystem ==
  note: M1
  Vs : Inport
  "E* " : Inport  Port=2
  Id : Inport  Port=3
  3M1/(2root2)1 : Gain  Gain=2*sqrt(2)/(3*sqrt(3))
  3M1/(2root2)2 : Gain  Gain=2*sqrt(2)/(3*sqrt(3))
  Divide : Product  Inputs=*/
  Fcn : Fcn  Expr=sqrt((u(1))^2 +((u(2))^2))
  Product : Product  RndMeth=Zero
  Ios : Outport
  wires:
  "E* "/1 -> Divide/2
  Vs/1 -> Fcn/1
  Fcn/1 -> Divide/1
  Divide/1 -> 3M1/(2root2)1/1
  3M1/(2root2)1/1 -> Product/1
  3M1/(2root2)2/1 -> Product/2
  Product/1 -> Ios/1
  Id/1 -> 3M1/(2root2)2/1

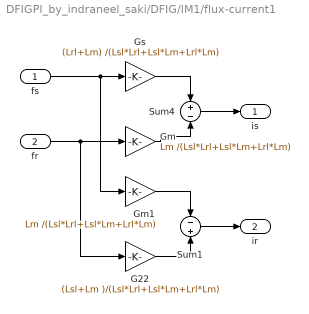
== system DFIGPI_by_indraneel_saki/DFIG/IM1/flux-current1 ==
  fs : Inport
  fr : Inport  Port=2
  G22 : Gain  Gain=(Lsl+Lm )/(Lsl*Lrl+Lsl*Lm+Lrl*Lm)  SaturateOnIntegerOverflow=on  OutDataTypeStr=Inherit: Same as input  ParamDataTypeStr=Inherit: Same as input
  Gm : Gain  Gain=Lm /(Lsl*Lrl+Lsl*Lm+Lrl*Lm)  SaturateOnIntegerOverflow=on  OutDataTypeStr=Inherit: Same as input  ParamDataTypeStr=Inherit: Same as input
  Gm1 : Gain  Gain=Lm /(Lsl*Lrl+Lsl*Lm+Lrl*Lm)  SaturateOnIntegerOverflow=on  OutDataTypeStr=Inherit: Same as input  ParamDataTypeStr=Inherit: Same as input
  Gs : Gain  Gain=(Lrl+Lm) /(Lsl*Lrl+Lsl*Lm+Lrl*Lm)  SaturateOnIntegerOverflow=on  OutDataTypeStr=Inherit: Same as input  ParamDataTypeStr=Inherit: Same as input
  Sum1 : Sum  Inputs=-+  SaturateOnIntegerOverflow=on  InputSameDT=on  OutDataTypeStr=Inherit: Same as first input
  Sum4 : Sum  Inputs=+-  SaturateOnIntegerOverflow=on  InputSameDT=on  OutDataTypeStr=Inherit: Same as first input
  is : Outport
  ir : Outport  Port=2
  wires:
  fs/1 -> Gs/1, Gm1/1
  Gs/1 -> Sum4/1
  fr/1 -> Gm/1, G22/1
  Gm/1 -> Sum4/2
  Sum4/1 -> is/1
  Gm1/1 -> Sum1/1
  G22/1 -> Sum1/2
  Sum1/1 -> ir/1

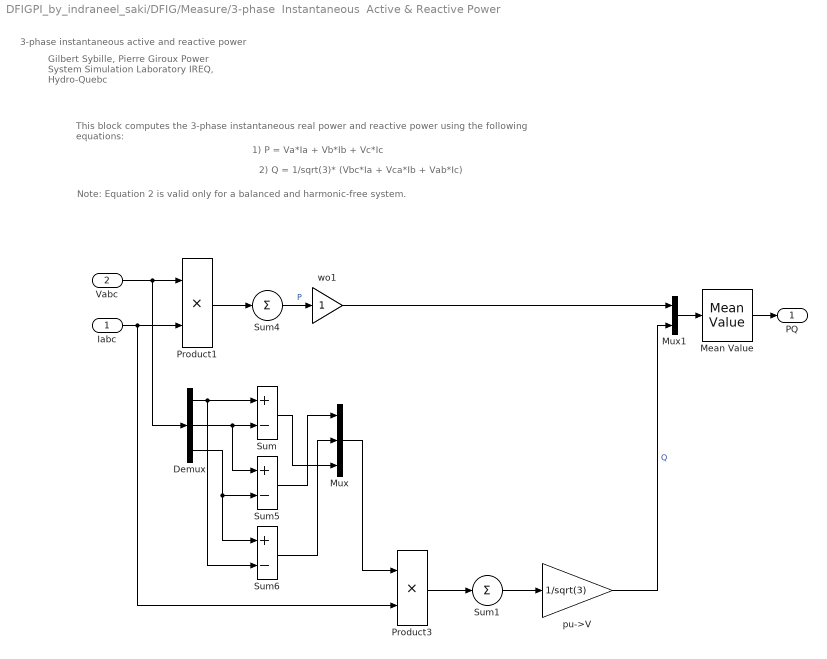
== system DFIGPI_by_indraneel_saki/DFIG/Measure/3-phase  Instantaneous  Active & Reactive Power ==
  note: 1) P = Va*Ia + Vb*Ib + Vc*Ic
  note: 2) Q = 1/sqrt(3)* (Vbc*Ia + Vca*Ib + Vab*Ic)
  note: This block computes the 3-phase instantaneous real power and reactive power using the following equations:
  note: Note: Equation 2 is valid only for a balanced and harmonic-free system.
  note: 3-phase instantaneous active and reactive power
  note: Gilbert Sybille, Pierre Giroux
      | Power System Simulation Laboratory
      | IREQ, Hydro-Quebc
  Iabc : Inport  PortDimensions=3
  Vabc : Inport  Port=2  PortDimensions=3
  Demux : Demux  Outputs=3
  Mean Value : powerlib_extras/Measurements/Mean Value  SystemSampleTime=-1  Period=1/60
      settings: SourceProductName=Simscape Electrical  SourceProductBaseCode=PS
  Mux : Mux  Inputs=3
  Mux1 : Mux  Inputs=2
  Product1 : Product  SaturateOnIntegerOverflow=on  InputSameDT=on  OutDataTypeStr=Inherit: Same as first input
  Product3 : Product  SaturateOnIntegerOverflow=on  InputSameDT=on  OutDataTypeStr=Inherit: Same as first input
  Sum : Sum  Inputs=+-  SaturateOnIntegerOverflow=on  InputSameDT=on  OutDataTypeStr=Inherit: Same as first input
  Sum1 : Sum  Inputs=1  SaturateOnIntegerOverflow=on  InputSameDT=on  OutDataTypeStr=Inherit: Same as first input
  Sum4 : Sum  Inputs=1  SaturateOnIntegerOverflow=on  InputSameDT=on  OutDataTypeStr=Inherit: Same as first input
  Sum5 : Sum  Inputs=+-  SaturateOnIntegerOverflow=on  InputSameDT=on  OutDataTypeStr=Inherit: Same as first input
  Sum6 : Sum  Inputs=+-  SaturateOnIntegerOverflow=on  InputSameDT=on  OutDataTypeStr=Inherit: Same as first input
  pu->V : Gain  Gain=1/sqrt(3)  SaturateOnIntegerOverflow=on  OutDataTypeStr=Inherit: Same as input  ParamDataTypeStr=Inherit: Same as input
  wo1 : Gain  SaturateOnIntegerOverflow=on  OutDataTypeStr=Inherit: Same as input  ParamDataTypeStr=Inherit: Same as input
  PQ : Outport
  wires:
  Sum1/1 -> pu->V/1
  Product3/1 -> Sum1/1
  Product1/1 -> Sum4/1
  Vabc/1 -> Product1/1, Demux/1
  Iabc/1 -> Product1/2, Product3/2
  Demux/1 -> Sum/1, Sum6/2
  Demux/2 -> Sum/2, Sum5/1
  Demux/3 -> Sum5/2, Sum6/1
  Sum/1 -> Mux/3
  Sum5/1 -> Mux/1
  Sum6/1 -> Mux/2
  Mux/1 -> Product3/1
  pu->V/1 -> Mux1/2  "Q"
  Mux1/1 -> Mean Value/1
  Sum4/1 -> wo1/1  "P"
  wo1/1 -> Mux1/1
  Mean Value/1 -> PQ/1

== system DFIGPI_by_indraneel_saki/DFIG/Measure/dq2ab  ==
  dq : Inport
  thetas : Inport  Port=2
  Fcn : Fcn  Expr=u(1)*cos(u(3))-u(2)*sin(u(3))
  Fcn1 : Fcn  Expr=u(1)*sin(u(3))+u(2)*cos(u(3))
  Mux3 : Mux  Inputs=2
  Mux4 : Mux  Inputs=2
  Mux5 : Mux  Inputs=2
  ab : Outport
  wires:
  Mux3/1 -> Fcn/1
  Mux4/1 -> Fcn1/1
  dq/1 -> Mux3/1, Mux4/1
  thetas/1 -> Mux3/2, Mux4/2
  Fcn1/1 -> Mux5/2
  Fcn/1 -> Mux5/1
  Mux5/1 -> ab/1

== system DFIGPI_by_indraneel_saki/DFIG/Measure/dq2ab 1 ==
  dq : Inport
  thetas : Inport  Port=2
  Fcn : Fcn  Expr=u(1)*cos(u(3))-u(2)*sin(u(3))
  Fcn1 : Fcn  Expr=u(1)*sin(u(3))+u(2)*cos(u(3))
  Mux3 : Mux  Inputs=2
  Mux4 : Mux  Inputs=2
  Mux5 : Mux  Inputs=2
  ab : Outport
  wires:
  Mux3/1 -> Fcn/1
  Mux4/1 -> Fcn1/1
  dq/1 -> Mux3/1, Mux4/1
  thetas/1 -> Mux3/2, Mux4/2
  Fcn1/1 -> Mux5/2
  Fcn/1 -> Mux5/1
  Mux5/1 -> ab/1

== system DFIGPI_by_indraneel_saki/DFIG/Measure/dq2ab 2 ==
  dq : Inport
  thetar : Inport  Port=2
  Fcn : Fcn  Expr=u(1)*cos(u(3))-u(2)*sin(u(3))
  Fcn1 : Fcn  Expr=u(1)*sin(u(3))+u(2)*cos(u(3))
  Mux3 : Mux  Inputs=2
  Mux4 : Mux  Inputs=2
  Mux5 : Mux  Inputs=2
  ab : Outport
  wires:
  Mux3/1 -> Fcn/1
  Mux4/1 -> Fcn1/1
  dq/1 -> Mux3/1, Mux4/1
  thetar/1 -> Mux3/2, Mux4/2
  Fcn1/1 -> Mux5/2
  Fcn/1 -> Mux5/1
  Mux5/1 -> ab/1

== system DFIGPI_by_indraneel_saki/DFIG/Measure/dq2ab 3 ==
  dq : Inport
  thetar : Inport  Port=2
  Fcn : Fcn  Expr=u(1)*cos(u(3))-u(2)*sin(u(3))
  Fcn1 : Fcn  Expr=u(1)*sin(u(3))+u(2)*cos(u(3))
  Mux3 : Mux  Inputs=2
  Mux4 : Mux  Inputs=2
  Mux5 : Mux  Inputs=2
  ab : Outport
  wires:
  Mux3/1 -> Fcn/1
  Mux4/1 -> Fcn1/1
  dq/1 -> Mux3/1, Mux4/1
  thetar/1 -> Mux3/2, Mux4/2
  Fcn1/1 -> Mux5/2
  Fcn/1 -> Mux5/1
  Mux5/1 -> ab/1
